simulink model "C1_sensor"  (Simulink 10.2)
settings: Solver=ode4  StartTime=0.0  StopTime=4  FixedStep=T_s*0.1  RelTol=1e-3
undefined symbols (not defined in the file): b_eq, beta_p, beta_v, g, i_rated, J_eq, k, L, L_l, m_l, N_e, N_opt, R, R_sh, T_s, tau_m_rated, theta_0, V_adc
libraries: simulink x1
settings Model: Creator=ioannis  LastModifiedBy=mfocchi
settings DataIOCC: SaveFormat=Dataset  SignalLoggingSaveFormat=Dataset
settings OptimizationCC: LifeSpan=auto
settings DebuggingCC: UnderspecifiedInitializationDetection=Simplified  MergeDetectMultiDrivingBlocksExec=error  FcnCallInpInsideContextMsg=error  SFUnexpectedBacktrackingDiag=error  SFNoUnconditionalDefaultTransitionDiag=error  SFExecutionAtInitializationDiag=warning
settings HardwareCC: ProdBitPerPointer=64  ProdBitPerSizeT=64  ProdBitPerPtrDiffT=64  ProdLargestAtomicFloat=Float  ProdIntDivRoundTo=Zero  ProdEndianess=LittleEndian  ProdWordSize=64  ProdHWDeviceType=Intel->x86-64 (Windows64)
settings ModelReferenceCC: PropagateSignalLabelsOutOfModel=on
settings SFSimCC: SimUseLocalCustomCode=on
settings RTWCC: RTWUseLocalCustomCode=on
settings CodeAppCC: StateflowObjectComments=off
settings GRTTargetCC: TargetLangStandard=C99 (ISO)  CombineOutputUpdateFcns=on  GRTInterface=off
settings ConfigComp: CovMetricSettings=dwe  CovSaveCumulativeToWorkspaceVar=off  CovSaveSingleToWorkspaceVar=off  CovExternalEMLEnable=on

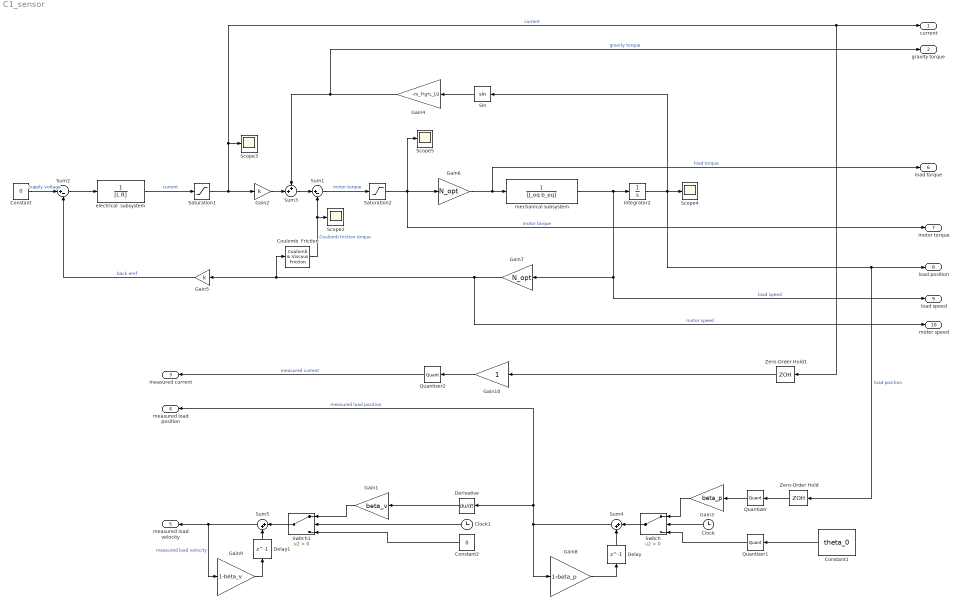
== system C1_sensor ==
  Clock : Clock
  Clock1 : Clock
  Constant : Constant  Value=0
  Constant1 : Constant  Value=theta_0
  Constant2 : Constant  Value=0
  Coulomb  Friction : simulink/Discontinuities/Coulomb & Viscous Friction  offset=tau_c  gain=0
  Delay : Delay  DelayLength=1  InitialCondition=0
  Delay1 : Delay  DelayLength=1  InitialCondition=0
  Derivative : Derivative
  Gain1 : Gain  Gain=beta_v
  Gain10 : Gain
  Gain2 : Gain  Gain=k
  Gain3 : Gain  Gain=beta_p
  Gain4 : Gain  Gain=-m_l*g*L_l/2
  Gain5 : Gain  Gain=k
  Gain6 : Gain  Gain=N_opt
  Gain7 : Gain  Gain=N_opt
  Gain8 : Gain  Gain=1-beta_p
  Gain9 : Gain  Gain=1-beta_v
  Integrator2 : Integrator  InitialCondition=theta_0
  Quantizer : Quantizer  QuantizationInterval=2*pi/(2^N_e)
  Quantizer1 : Quantizer  QuantizationInterval=2*pi/(2^N_e)
  Quantizer2 : Quantizer  QuantizationInterval=V_adc/R_sh/(2^N_e)
  Saturation1 : Saturate  UpperLimit=i_rated  LowerLimit=-i_rated
  Saturation2 : Saturate  UpperLimit=tau_m_rated  LowerLimit=-tau_m_rated
  Scope{2..5} (4 alike) : Scope
  Sin : Trigonometry
  Sum1 : Sum  Inputs=|+-
  Sum2 : Sum  Inputs=|+-
  Sum3 : Sum  Inputs=++|
  Sum4 : Sum  Inputs=|++
  Sum5 : Sum  Inputs=|++
  Switch : Switch  Criteria=u2 > Threshold
  Switch1 : Switch  Criteria=u2 > Threshold
  Zero-Order Hold : ZeroOrderHold  SampleTime=T_s
  Zero-Order Hold1 : ZeroOrderHold  SampleTime=T_s
  electrical  subsystem : TransferFcn  Denominator=[L R]
  mechanical subsystem : TransferFcn  Denominator=[J_eq b_eq]
  current : Outport
  gravity torque : Outport  Port=2
  measured current : Outport  Port=3
  measured load position : Outport  Port=4
  measured load velocity : Outport  Port=5
  load torque : Outport  Port=6
  motor torque : Outport  Port=7
  load position : Outport  Port=8
  load speed : Outport  Port=9
  motor speed : Outport  Port=10
  wires:
  Gain7/1 -> motor speed/1, Coulomb  Friction/1, Gain5/1  "motor speed"
  Constant/1 -> Sum2/1  "Supply voltage"
  mechanical subsystem/1 -> Gain7/1, load speed/1, Integrator2/1  "load speed"
  Sum2/1 -> electrical  subsystem/1
  Coulomb  Friction/1 -> Sum1/2, Scope2/1  "Coulomb friction torque"
  electrical  subsystem/1 -> Saturation1/1  "current"
  Saturation1/1 -> Zero-Order Hold1/1, current/1, Scope3/1, Gain2/1  "current"
  Sum1/1 -> Saturation2/1  "motor torque"
  Saturation2/1 -> motor torque/1, Scope5/1, Gain6/1  "motor torque"
  Sin/1 -> Gain4/1
  Gain2/1 -> Sum3/2
  Sum3/1 -> Sum1/1
  Gain4/1 -> gravity torque/1, Sum3/1  "gravity torque"
  Gain5/1 -> Sum2/2  "back emf"
  Integrator2/1 -> Sin/1, Zero-Order Hold/1, load position/1, Scope4/1  "load position"
  Gain6/1 -> load torque/1, mechanical subsystem/1  "load torque"
  Delay1/1 -> Sum5/2
  Gain8/1 -> Delay/1
  Gain3/1 -> Switch/1
  Switch/1 -> Sum4/1
  Sum4/1 -> measured load position/1, Derivative/1, Gain8/1  "measured load position"
  Constant2/1 -> Switch1/3
  Derivative/1 -> Gain1/1
  Gain10/1 -> Quantizer2/1
  Quantizer/1 -> Gain3/1
  Clock/1 -> Switch/2
  Switch1/1 -> Sum5/1
  Clock1/1 -> Switch1/2
  Constant1/1 -> Quantizer1/1
  Quantizer2/1 -> measured current/1  "measured current"
  Quantizer1/1 -> Switch/3
  Gain9/1 -> Delay1/1
  Gain1/1 -> Switch1/1
  Delay/1 -> Sum4/2
  Sum5/1 -> Gain9/1, measured load velocity/1  "measured load velocity"
  Zero-Order Hold/1 -> Quantizer/1
  Zero-Order Hold1/1 -> Gain10/1
